simulink model "lab2_schema_fig21"  (R2023b)
settings: Solver=ode45  StartTime=0.0  StopTime=300  RelTol=1e-3
settings Model: Creator=Daniela  LastModifiedBy=Daniela

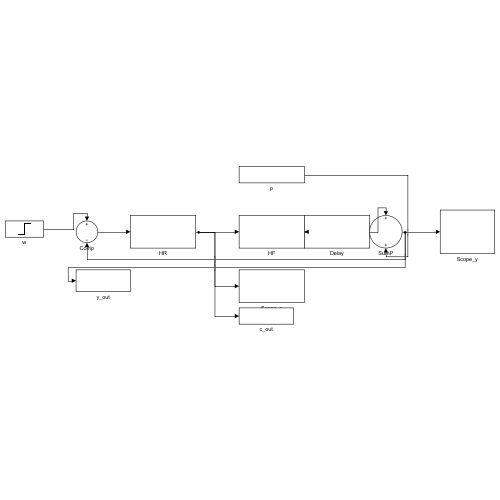
[thumbnail: Simulink's stored preview of the top-level diagram]
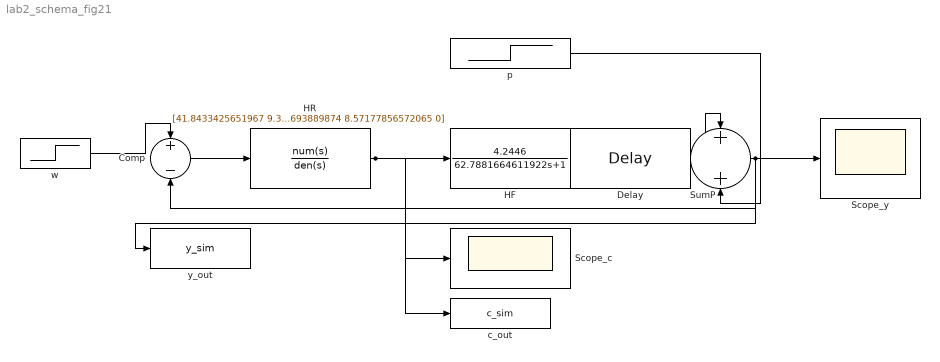
== system lab2_schema_fig21 ==
  Comp : Sum  Inputs=+-
  Delay : TransportDelay  DelayTime=8.5718
  HF : TransferFcn  Numerator=4.2446  Denominator=[62.7881664611922 1]
  HR : TransferFcn  Numerator=[41.8433425651967 9.31927304056271 1.03543250281373]  Denominator=[3.6737693889874 8.57177856572065 0]
  Scope_c : Scope
  Scope_y : Scope
  SumP : Sum
  c_out : ToWorkspace  VariableName=c_sim  SampleTime=-1
  p : Step  Time=0  After=0  SampleTime=0
  w : Step  Time=0  SampleTime=0
  y_out : ToWorkspace  VariableName=y_sim  SampleTime=-1
  wires:
  w/1 -> Comp/1
  Comp/1 -> HR/1
  HR/1 -> HF/1, Scope_c/1, c_out/1
  HF/1 -> Delay/1
  Delay/1 -> SumP/1
  p/1 -> SumP/2
  SumP/1 -> Scope_y/1, y_out/1, Comp/2
